simulink model "mrac_classic"  (R2023b)
settings: Solver=ode5  StartTime=0.0  StopTime=120  FixedStep=0.001  RelTol=1e-3
settings Model: Creator=merve  LastModifiedBy=hiobj
settings DataIOCC: ReturnWorkspaceOutputs=off

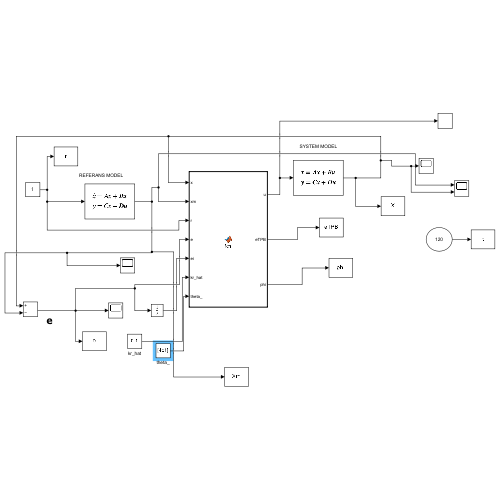
[thumbnail: Simulink's stored preview of the top-level diagram]
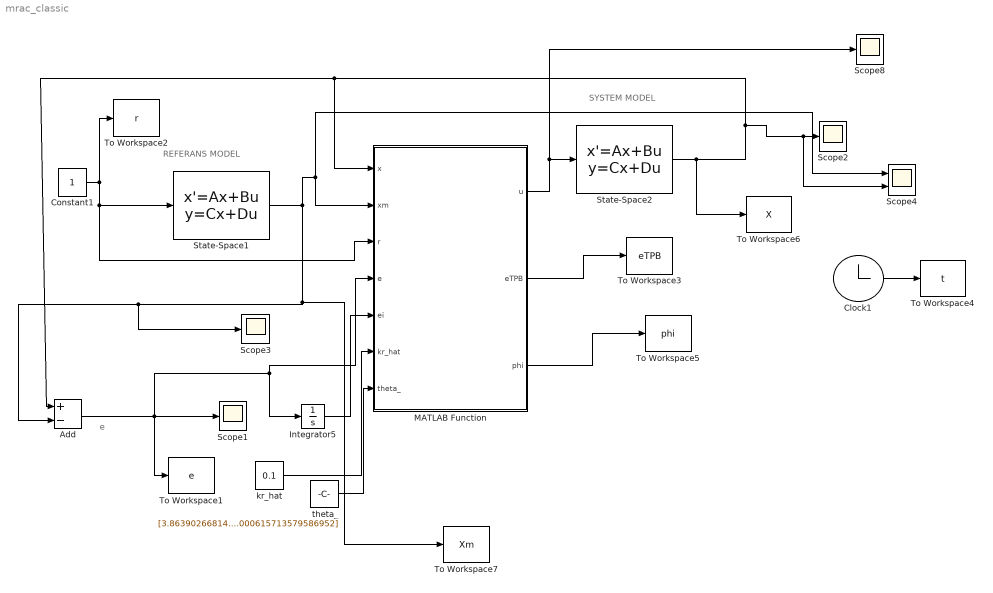
== system mrac_classic ==
  note: e
  note: REFERANS MODEL
  note: SYSTEM MODEL
  Add : Sum  Inputs=+-
  Clock1 : Clock
  Constant1 : Constant  SampleTime=0.001
  Integrator5 : Integrator
  MATLAB Function : MATLAB Function  TreatAsAtomicUnit=on
  Scope{1..3,8} (4 alike) : Scope
  Scope4 : Scope  NumInputPorts=2
  State-Space1 : StateSpace  A=[0 1;-4 -4]  B=[0;4]  C=[1 0;0 1]  D=[0;0]  InitialCondition=0
  State-Space2 : StateSpace  A=[0 1;1 0]  B=[0;1]  C=[1 0;0 1]  D=[0;0]  InitialCondition=0
  To Workspace1 : ToWorkspace  VariableName=e  SampleTime=-1
  To Workspace2 : ToWorkspace  VariableName=r  SampleTime=-1
  To Workspace3 : ToWorkspace  VariableName=eTPB  SampleTime=-1
  To Workspace4 : ToWorkspace  VariableName=t  SampleTime=-1
  To Workspace5 : ToWorkspace  VariableName=phi  SampleTime=-1
  To Workspace6 : ToWorkspace  VariableName=X  SampleTime=-1
  To Workspace7 : ToWorkspace  VariableName=Xm  SampleTime=-1
  kr_hat : Constant  Value=0.1  SampleTime=0.001
  theta_ : Constant  Value=[3.86390266814324e-05;0.000154346322729147;0.000346808616437119;0.000615713579586952]  VectorParams1D=off  SampleTime=0.001
  wires:
  Constant1/1 -> To Workspace2/1, State-Space1/1, MATLAB Function/3(r)
  State-Space2/1 -> To Workspace6/1, Scope4/2, Scope2/1, MATLAB Function/1(x), Add/1
  Add/1 -> To Workspace1/1, Integrator5/1, MATLAB Function/4(e), Scope1/1
  MATLAB Function/1(u) -> Scope8/1, State-Space2/1
  Clock1/1 -> To Workspace4/1
  State-Space1/1 -> Scope4/1, MATLAB Function/2(xm), To Workspace7/1, Scope3/1, Add/2
  Integrator5/1 -> MATLAB Function/5(ei)
  MATLAB Function/2(eTPB) -> To Workspace3/1
  kr_hat/1 -> MATLAB Function/6(kr_hat)
  theta_/1 -> MATLAB Function/7(theta_)
  MATLAB Function/3(phi) -> To Workspace5/1

== matlab function mrac_classic/MATLAB Function ==
  settings: updateMethod=DISCRETE
  data: x input; u output; xm input; r input; e input; ei input; eTPB output; kr_hat input; theta_ input; phi output
function [u, eTPB, phi] = fcn(x, xm, r, e, ei, kr_hat, theta_)


          P=[0.5,0.27;0.27,0.46];

    % gamma_Kr = 1;
    % gamma_kr = 100;
    % gamma_theta = 1;
    %   3.5943    4.7982
    % 4.7982    9.9342
       % P = [2.4, 2.1;2.1, 3.359];
      % P=[1.7,0.05331;0.5331,0.1457];
    B = [0; 1];
% P = [3.6, 4.7;4.7, 9.9];
    phi = [x; ei];        % [3x1]
    eTPB = e' * P * B;    % skalar

    % persistent theta_
    % if isempty(theta_)
    %     theta_ = zeros(4,1);   % adaptif genişletilmiş parametreler
    % end
    % if isempty(kr_hat)
    %     kr_hat = 0;            % tahmin edilen kr
    % end

    % % Proportional + integral adaptasyon
    % kr_dot = -gamma_kr * r * eTPB;  
    % kr_hat = kr_hat + 0.001 * kr_dot;

    % Kontrol sinyalinin PI-AM versiyonu
    % theta_dot = -gamma_theta * eTPB * phi;
    % theta_ = theta_ + 0.001 * theta_dot;

    % Kr sabit (bu örnekte güncellenmiyor)
    Kr = [-1; -1.4];  % Tezdeki uyumlu sabit değer
          Kr1=[-0.23;-0.8];
          Kr3=[-0.94;-1.6];
    % Final kontrol sinyali
    u = Kr' * x + kr_hat * r + theta_' * phi;

   
end
